simulink model "test_vacc_pkt_10_1"  (Simulink 7.2)
settings: Solver=ode45  StartTime=0.0  StopTime=90000  RelTol=1e-3
libraries: xbsIndex_r4 x802, xps_library x17, casper_library_misc x10, xbsReplacements_r4 x9
(part 1 of 6)
settings Model: Creator=Jason Manley  LastModifiedBy=root
settings OptimizationCC: InitFltsAndDblsToZero=on
settings DebuggingCC: SaveWithParameterizedLinksMsg=none  SignalResolutionControl=TryResolveAllWithWarning  MultiTaskDSMMsg=warning  MultiTaskCondExecSysMsg=none  StrictBusMsg=None
settings RTWCC: IncludeERTFirstTime=on
settings GRTTargetCC: TargetFcnLib=ansi_tfl_tmw.mat

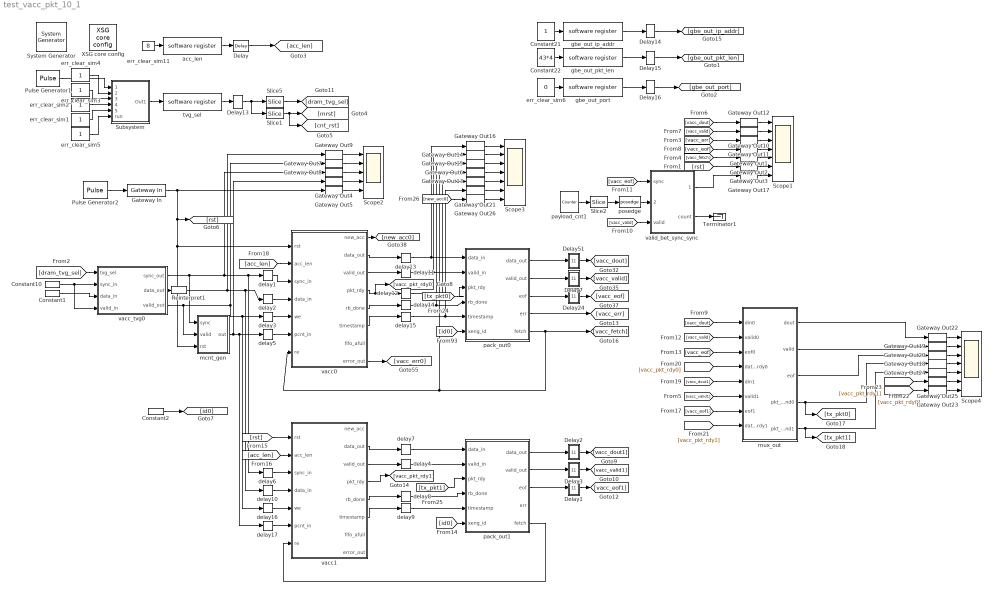
== system test_vacc_pkt_10_1 ==
  " System Generator" : xbsIndex_r4/ System Generator  Tag=genX  SystemSampleTime=-1  xilinxfamily=virtex5  part=xc5vlx110t  speed=-1  package=ff1136  synthesis_tool=XST  clock_wrapper=Clock Enables  directory=./test_vacc_pkt_10_1/sysgen  testbench=off  simulink_period=1  sysclk_period=5  dcm_input_clock_period=100  incr_netlist=off  trim_vbits=Everywhere in SubSystem  dbl_ovrd=According to Block Masks  core_generation=According to Block Masks  run_coregen=off  deprecated_control=off  eval_field=0  block_type=sysgen
      settings: block_version=10.1.3
  Constant1 : xbsIndex_r4/Constant  arith_type=Unsigned  const=0  n_bits=32  bin_pt=0  explicit_period=on  period=1  equ=P=C  opselect=C  inp2=PCIN>>17  opr=+  inp1=P  carry=CIN  dbl_ovrd=off  block_type=constant
  Constant10 : xbsIndex_r4/Constant  arith_type=Boolean  const=0  n_bits=1  bin_pt=0  explicit_period=on  period=1  equ=P=C  opselect=C  inp2=PCIN>>17  opr=+  inp1=P  carry=CIN  dbl_ovrd=off  block_type=constant
  Constant2 : xbsIndex_r4/Constant  arith_type=Unsigned  const=0  n_bits=4  bin_pt=0  explicit_period=on  period=1  equ=P=C  opselect=C  inp2=PCIN>>17  opr=+  inp1=P  carry=CIN  dbl_ovrd=off  block_type=constant
  Constant21 : Constant  OutDataType=sfix(16)  OutScaling=2^0
  Constant22 : Constant  Value=43*4  OutDataType=sfix(16)  OutScaling=2^0
  Delay : xbsIndex_r4/Delay  en=off  latency=1  dbl_ovrd=off  reg_retiming=on  block_type=delay
  Delay1 : Subsystem  AncestorBlock=casper_library/Delays/pipeline  mask(pipeline){latency=2}
      mask help:
      | An explicitly laid-out delay line to avoid mapping to SRL16s
      | for use in pipelining to help achieve timing closure.
      mask init:
      | pipeline_init(gcb, 'latency', latency);
      mask Display:
      | port_label('input', 1, 'd');
      | port_label('output', 1, 'q');
      | disp(['Z^-', num2str(latency)]);
  Delay{13..16} (4 alike) : xbsIndex_r4/Delay  en=off  latency=2  dbl_ovrd=off  reg_retiming=on  block_type=delay
      settings: xl_area=[0, 0, 0, 0, 0, 0, 0]
  Delay2 : Subsystem  AncestorBlock=casper_library/Delays/pipeline  mask(pipeline){latency=2}
      mask help:
      | An explicitly laid-out delay line to avoid mapping to SRL16s
      | for use in pipelining to help achieve timing closure.
      mask init:
      | pipeline_init(gcb, 'latency', latency);
      mask Display:
      | port_label('input', 1, 'd');
      | port_label('output', 1, 'q');
      | disp(['Z^-', num2str(latency)]);
  Delay24 : Subsystem  AncestorBlock=casper_library/Delays/pipeline  mask(pipeline){latency=2}
      mask help:
      | An explicitly laid-out delay line to avoid mapping to SRL16s
      | for use in pipelining to help achieve timing closure.
      mask init:
      | pipeline_init(gcb, 'latency', latency);
      mask Display:
      | port_label('input', 1, 'd');
      | port_label('output', 1, 'q');
      | disp(['Z^-', num2str(latency)]);
  Delay3 : Subsystem  AncestorBlock=casper_library/Delays/pipeline  mask(pipeline){latency=2}
      mask help:
      | An explicitly laid-out delay line to avoid mapping to SRL16s
      | for use in pipelining to help achieve timing closure.
      mask init:
      | pipeline_init(gcb, 'latency', latency);
      mask Display:
      | port_label('input', 1, 'd');
      | port_label('output', 1, 'q');
      | disp(['Z^-', num2str(latency)]);
  Delay51 : Subsystem  AncestorBlock=casper_library/Delays/pipeline  mask(pipeline){latency=2}
      mask help:
      | An explicitly laid-out delay line to avoid mapping to SRL16s
      | for use in pipelining to help achieve timing closure.
      mask init:
      | pipeline_init(gcb, 'latency', latency);
      mask Display:
      | port_label('input', 1, 'd');
      | port_label('output', 1, 'q');
      | disp(['Z^-', num2str(latency)]);
  Delay7 : Subsystem  AncestorBlock=casper_library/Delays/pipeline  mask(pipeline){latency=2}
      mask help:
      | An explicitly laid-out delay line to avoid mapping to SRL16s
      | for use in pipelining to help achieve timing closure.
      mask init:
      | pipeline_init(gcb, 'latency', latency);
      mask Display:
      | port_label('input', 1, 'd');
      | port_label('output', 1, 'q');
      | disp(['Z^-', num2str(latency)]);
  Gateway In : xbsIndex_r4/Gateway In  arith_type=Boolean  n_bits=16  bin_pt=14  quantization="Round  (unbiased: +/- Inf)"  overflow=Saturate  period=1  dbl_ovrd=off  timing_constraint=None  locs_specified=off  LOCs={}  hdl_port=on  block_type=gatewayin
      settings: infoedit="Gateway in block.  Converts inputs of type Simulink integer, double and fixed point to  Xilinx fixed point type.<br><br>Hardware notes:  In hardware these blocks become top level input ports."  block_version=11.4
  Gateway Out{1..26} (26 alike) : xbsIndex_r4/Gateway Out  hdl_port=off  timing_constraint=None  locs_specified=off  LOCs={}  block_type=gatewayout
      settings: infoedit="Gateway out block.  Converts Xilinx fixed point inputs into ouputs of type Simulink integer, double, or fixed point.<P><P>Hardware notes:  In hardware these blocks become top level output ports or are discarded, depending on how they are configured."  xl_area=[0, 0, 0, 0, 0, 0, 0]  block_version=10.1.3
  Pulse Generator1 : DiscretePulseGenerator  Period=4*100*80  PhaseDelay=-4*100*80 + 3
  Pulse Generator2 : DiscretePulseGenerator  Period=8*100*80  PhaseDelay=-2*100*10 + 1
  Reinterpret1 : xbsIndex_r4/Reinterpret  force_arith_type=on  arith_type="Signed  (2's comp)"  force_bin_pt=on  bin_pt=0  block_type=reinterpret
      settings: infoedit="Changes signal type without altering the binary representation.   You can changed the signal between signed and unsigned, and relocate the binary point.<P><P>Hardware notes: In hardware this block costs nothing.<P><P>Example:  Suppose the input is 6 bits wide, signed, with 2 fractional bits, and the output is forced to unsigned with 0 fractional bits.  Then an input of -2.0 (1110.00 in binary 2's complement) becomes an output of 56 (111000 in binary)."  block_version=10.1.3
  Scope1 : Scope  NumInputPorts=7
      settings: YMin=0~0~-1~0~0~0~0  YMax=2.5e+21~1~1~1~1~1~40  SaveName=ScopeData7
  Scope2 : Scope  NumInputPorts=5
      settings: YMin=0~0~0~0~0  YMax=100~1~1~35000~1  SaveName=ScopeData8
  Scope3 : Scope  NumInputPorts=7
      settings: YMin=0~0~0~0~0~0~0  YMax=800~1~1~1~1~17500~1  SaveName=ScopeData10
  Scope4 : Scope  NumInputPorts=7
      settings: YMin=0~0~0~-1~0~-1~0  YMax=1e+19~1~1~1~1~1~1  SaveName=ScopeData11
  Slice1 : xbsIndex_r4/Slice  nbits=1  boolean_output=on  mode=Lower Bit Location + Width  bit1=0  base1=MSB of Input  bit0=31  base0=LSB of Input  dbl_ovrd=off  block_type=slice
      settings: infoedit="Extracts a given range of bits from each input sample and presents it at the output.  The output type is ordinarily unsigned with binary point at zero, but can be Boolean when the slice is one bit wide.<P><P>Hardware notes: In hardware this block costs nothing."  block_version=10.1.3
  Slice2 : xbsIndex_r4/Slice  nbits=1  boolean_output=on  mode=Upper Bit Location + Width  bit1=0  base1=MSB of Input  bit0=1  base0=LSB of Input  dbl_ovrd=off  block_type=slice
      settings: infoedit="Extracts a given range of bits from each input sample and presents it at the output.  The output type is ordinarily unsigned with binary point at zero, but can be Boolean when the slice is one bit wide.<P><P>Hardware notes: In hardware this block costs nothing."  block_version=10.1.3
  Slice5 : xbsIndex_r4/Slice  nbits=6  boolean_output=off  mode=Lower Bit Location + Width  bit1=0  base1=MSB of Input  bit0=9  base0=LSB of Input  dbl_ovrd=off  block_type=slice
      settings: infoedit="Extracts a given range of bits from each input sample and presents it at the output.  The output type is ordinarily unsigned with binary point at zero, but can be Boolean when the slice is one bit wide.<P><P>Hardware notes: In hardware this block costs nothing."  block_version=10.1.3
  Subsystem : Subsystem
  Terminator1 : Terminator
  XSG core config : xps_library/XSG core config  Tag=xps:xsg  SystemSampleTime=-1  hw_sys=iBOB  ibob_linux=off  clk_src=sys_clk  iBOB_clk_src=sys_clk  BEE2_ctrl_clk_src=sys_clk  BEE2_usr_clk_src=sys_clk  ROACH_clk_src=arb_clk  ROACH2_clk_src=adc0_clk  CORR_clk_src=sys_clk  gpio_clk_io_group=iBOB:sma  gpio_clk_bit_index=0  clk_rate=100  sample_period=1  synthesis_tool=XST  mpc_type=powerpc405
  acc_len : xps_library/software register  Tag=xps:sw_reg  SystemSampleTime=-1  io_dir=From Processor  arith_type=Unsigned  bitwidth=32  bin_pt=0  sample_period=1  gw_name=test_vacc_pkt_10_1_acc_len_user_data_out
      link override qdr_vacc_tvg_sel_user_data_out: arith_type=Unsigned  n_bits=32  bin_pt=0  period=1
      link override test_d_v_p_10_1_new_packet_format_acc_len_user_data_out: arith_type=Unsigned  n_bits=32  bin_pt=0  period=1
      link override test_qdr_vacc_acc_len_user_data_out: arith_type=Unsigned  n_bits=32  bin_pt=0  period=1
      link override test_qdr_vacc_tvg_sel_user_data_out: arith_type=Unsigned  n_bits=32  bin_pt=0  period=1
      link override test_vacc_10_1_new_pkt_form_acc_len_user_data_out: arith_type=Unsigned  n_bits=32  bin_pt=0  period=1
      link override test_vacc_pkt_10_1_acc_len_user_data_out: arith_type=Unsigned  n_bits=32  bin_pt=0  period=1
  delay{1..3,5..6,10,16..17} (8 alike) : xbsIndex_r4/Delay  en=off  latency=2  dbl_ovrd=off  reg_retiming=on  block_type=delay
  delay{4,7..9,11..15} (9 alike) : xbsIndex_r4/Delay  en=off  latency=1  dbl_ovrd=off  reg_retiming=on  block_type=delay
  err_clear_sim{1..5} (5 alike) : Constant  OutDataType=sfix(16)  OutScaling=2^0
  err_clear_sim11 : Constant  Value=8  OutDataType=sfix(16)  OutScaling=2^0
  err_clear_sim6 : Constant  Value=0  OutDataType=sfix(16)  OutScaling=2^0
  gbe_out_ip_addr : xps_library/software register  Tag=xps:sw_reg  SystemSampleTime=-1  io_dir=From Processor  arith_type=Unsigned  bitwidth=32  bin_pt=0  sample_period=1  gw_name=test_vacc_pkt_10_1_gbe_out_ip_addr_user_data_out
      link override test_d_v_p_10_1_new_packet_format_gbe_out_ip_addr_user_data_out: arith_type=Unsigned  n_bits=32  bin_pt=0  period=1
      link override test_d_v_p_10_1_new_packet_format_out_ip_addr_user_data_out: arith_type=Unsigned  n_bits=32  bin_pt=0  period=1
      link override test_vacc_10_1_new_pkt_form_gbe_out_ip_addr_user_data_out: arith_type=Unsigned  n_bits=32  bin_pt=0  period=1
      link override test_vacc_pkt_10_1_gbe_out_ip_addr_user_data_out: arith_type=Unsigned  n_bits=32  bin_pt=0  period=1
  gbe_out_pkt_len : xps_library/software register  Tag=xps:sw_reg  SystemSampleTime=-1  io_dir=From Processor  arith_type=Unsigned  bitwidth=32  bin_pt=0  sample_period=1  gw_name=test_vacc_pkt_10_1_gbe_out_pkt_len_user_data_out
      link override test_d_v_p_10_1_new_packet_format_gbe_out_pkt_len_user_data_out: arith_type=Unsigned  n_bits=32  bin_pt=0  period=1
      link override test_d_v_p_10_1_new_packet_format_pkt_len_user_data_out: arith_type=Unsigned  n_bits=32  bin_pt=0  period=1
      link override test_vacc_10_1_new_pkt_form_gbe_out_pkt_len_user_data_out: arith_type=Unsigned  n_bits=32  bin_pt=0  period=1
      link override test_vacc_pkt_10_1_gbe_out_pkt_len_user_data_out: arith_type=Unsigned  n_bits=32  bin_pt=0  period=1
  gbe_out_port : xps_library/software register  Tag=xps:sw_reg  SystemSampleTime=-1  io_dir=From Processor  arith_type=Unsigned  bitwidth=32  bin_pt=0  sample_period=1  gw_name=test_vacc_pkt_10_1_gbe_out_port_user_data_out
      link override test_d_v_p_10_1_new_packet_format_gbe_out_port_user_data_out: arith_type=Unsigned  n_bits=32  bin_pt=0  period=1
      link override test_vacc_10_1_new_pkt_form_gbe_out_port_user_data_out: arith_type=Unsigned  n_bits=32  bin_pt=0  period=1
      link override test_vacc_pkt_10_1_gbe_out_port_user_data_out: arith_type=Unsigned  n_bits=32  bin_pt=0  period=1
  mcnt_gen : Subsystem  mask(sample_and_hold){period=100}
      mask prompts: period "Sample period (clocks)"
      mask help: This block will sample an input signal at a user specified rate and hold the value on the output.
  mux_out : Subsystem  mask{idle_clks=100}
      mask prompts: idle_clks "Rate control. Idle clocks between packets"
      mask init:
      | idle_clks_bits = ceil(log2(idle_clks));
      settings: AttributesFormatString=|
      | Payload Len: 32
      | FIFO latencies: 4.
  pack_out0 : Subsystem  mask(pkt_pack_mask){vector_len=100, heap_len=2000, fifo_latency=2, spead_msw=64, spead_lsw=40, spead_item=6144, pkt_bits=5}
      mask prompts: vector_len "vector length"; heap_len "System heap size"; fifo_latency "Fifo Latency"; spead_msw "SPEAD flavour (MSw)"; spead_lsw "SPEAD flavour (LSw)"; spead_item "SPEAD item number"; pkt_bits "desired payload length (2^?) 64-bit words"
      mask help:
      | This block generates packets from a datastream.
      |
      | Packets are created with a fixed header followed by a user-specified number of 64-bit options.
      |
      | Requires a 64-bit data stream.
      |
      | See the documentation for further details.
      mask init:
      | vector_bits = ceil(log2(vector_len));
      | pkt_len=2^(pkt_bits);
  pack_out1 : Subsystem  mask(pkt_pack_mask){vector_len=100, heap_len=2000, fifo_latency=2, spead_msw=64, spead_lsw=40, spead_item=6144, pkt_bits=5}
      mask prompts: vector_len "vector length"; heap_len "System heap size"; fifo_latency "Fifo Latency"; spead_msw "SPEAD flavour (MSw)"; spead_lsw "SPEAD flavour (LSw)"; spead_item "SPEAD item number"; pkt_bits "desired payload length (2^?) 64-bit words"
      mask help:
      | This block generates packets from a datastream.
      |
      | Packets are created with a fixed header followed by a user-specified number of 64-bit options.
      |
      | Requires a 64-bit data stream.
      |
      | See the documentation for further details.
      mask init:
      | vector_bits = ceil(log2(vector_len));
      | pkt_len=2^(pkt_bits);
  payload_cnt1 : xbsIndex_r4/Counter  cnt_type=Free Running  cnt_to=0  operation=Up  start_count=0  cnt_by_val=1  arith_type=Unsigned  n_bits=12  bin_pt=0  load_pin=off  rst=off  en=off  explicit_period=on  period=1  dbl_ovrd=off  use_behavioral_HDL=off  implementation=Fabric  use_rpm=on  block_type=counter
      settings: xl_area=[0, 0, 0, 0, 0, 0, 0]
  posedge : casper_library_misc/posedge  Tag=Rising Edge Detector  SystemSampleTime=-1
  tvg_sel : xps_library/software register  Tag=xps:sw_reg  SystemSampleTime=-1  io_dir=From Processor  arith_type=Unsigned  bitwidth=32  bin_pt=0  sample_period=1  gw_name=test_vacc_pkt_10_1_tvg_sel_user_data_out
      link override test_d_v_p_10_1_new_packet_format_tvg_sel_user_data_out: arith_type=Unsigned  n_bits=32  bin_pt=0  period=1
      link override test_vacc_10_1_new_pkt_form_tvg_sel_user_data_out: arith_type=Unsigned  n_bits=32  bin_pt=0  period=1
      link override test_vacc_pkt_10_1_tvg_sel_user_data_out: arith_type=Unsigned  n_bits=32  bin_pt=0  period=1
  vacc0 : Subsystem  mask{which_qdr=qdr0, vector_len=100}
      mask prompts: which_qdr "QDR"
      mask help: Hardcoded for X engines with a demux of 8!
      mask init:
      | set_param([gcb, '/qv'], 'which_qdr', which_qdr);
      | fmtstr = sprintf('Vector Length: %d', vector_len);
      | set_param(gcb, 'AttributesFormatString', fmtstr);
      settings: AttributesFormatString=Vector Length: 100
      mask StyleString: popup(qdr0|qdr1),edit
  vacc1 : Subsystem  mask{which_qdr=qdr0, vector_len=100}
      mask prompts: which_qdr "QDR"
      mask help: Hardcoded for X engines with a demux of 8!
      mask init:
      | set_param([gcb, '/qv'], 'which_qdr', which_qdr);
      | fmtstr = sprintf('Vector Length: %d', vector_len);
      | set_param(gcb, 'AttributesFormatString', fmtstr);
      settings: AttributesFormatString=Vector Length: 100
      mask StyleString: popup(qdr0|qdr1),edit
  vacc_tvg0 : Subsystem  AncestorBlock=casper_library/Accumulators/vacc_tvg  mask{len=100}
      mask prompts: len "Number of Vectors"
      mask init:
      | fmtstr = sprintf('Vector Length: %d', len);
      | set_param(gcb, 'AttributesFormatString', fmtstr);
      settings: AttributesFormatString=Vector Length: 100
  valid_bet_sync_sync : Subsystem
  wires:
  tvg_sel/1 -> Delay13/1
  Slice5/1 -> [dram_tvg_sel]
  err_clear_sim1/1 -> Subsystem/5(data_sel)
  err_clear_sim2/1 -> Subsystem/4(valid_sel)
  err_clear_sim3/1 -> Subsystem/3(inj_vector)
  err_clear_sim4/1 -> Subsystem/2(inj_counter)
  Subsystem/1(Out1) -> tvg_sel/1
  Pulse Generator1/1 -> Subsystem/1(new_acc)
  err_clear_sim5/1 -> Subsystem/6(run)
  Constant22/1 -> gbe_out_pkt_len/1
  Constant21/1 -> gbe_out_ip_addr/1
  gbe_out_ip_addr/1 -> Delay14/1
  gbe_out_pkt_len/1 -> Delay15/1
  Slice1/1 -> [mrst], [cnt_rst]
  acc_len/1 -> Delay/1
  err_clear_sim11/1 -> acc_len/1
  err_clear_sim6/1 -> gbe_out_port/1
  gbe_out_port/1 -> Delay16/1
  Delay13/1 -> Slice5/1, Slice1/1
  Delay14/1 -> [gbe_out_ip_addr]
  Delay15/1 -> [gbe_out_pkt_len]
  Delay16/1 -> [gbe_out_port]
  pack_out0/3(eof) -> Delay24/1(d)
  pack_out0/1(data_out) -> Delay51/1(d)
  pack_out0/2(valid_out) -> Delay7/1(d)
  Gateway In/1 -> Gateway Out5/1, mcnt_gen/3(rst), vacc0/1(rst), [rst]
  Delay51/1(q) -> [vacc_dout]
  Delay7/1(q) -> [vacc_valid]
  Delay24/1(q) -> [vacc_eof]
  vacc_tvg0/1(sync_out) -> Gateway Out8/1, delay1/1, delay6/1, mcnt_gen/1(sync)
  vacc_tvg0/2(data_out) -> Reinterpret1/1
  vacc_tvg0/3(valid_out) -> Gateway Out7/1, delay3/1, delay16/1, mcnt_gen/2(valid)
  Reinterpret1/1 -> Gateway Out9/1, delay2/1, delay10/1
  Delay/1 -> [acc_len]
  [dram_tvg_sel] -> vacc_tvg0/1(tvg_sel)
  Constant10/1 -> vacc_tvg0/2(sync_in), vacc_tvg0/4(valid_in)
  Constant1/1 -> vacc_tvg0/3(data_in)
  Gateway Out5/1 -> Scope2/5
  Gateway Out4/1 -> Scope2/4
  Gateway Out9/1 -> Scope2/1
  Gateway Out7/1 -> Scope2/2
  Gateway Out8/1 -> Scope2/3
  Gateway Out3/1 -> Scope1/6
  Gateway Out2/1 -> Scope1/5
  Gateway Out1/1 -> Scope1/4
  Gateway Out12/1 -> Scope1/1
  Gateway Out10/1 -> Scope1/2
  Gateway Out11/1 -> Scope1/3
  [vacc_dout] -> Gateway Out12/1
  [vacc_valid] -> Gateway Out10/1
  [vacc_eof] -> Gateway Out1/1
  Gateway Out13/1 -> Scope3/5
  Gateway Out6/1 -> Scope3/4
  Gateway Out16/1 -> Scope3/1
  Gateway Out14/1 -> Scope3/2
  Gateway Out15/1 -> Scope3/3
  valid_bet_sync_sync/2(count) -> Terminator1/1
  [vacc_valid] -> valid_bet_sync_sync/3(valid)
  [vacc_eof] -> valid_bet_sync_sync/1(sync)
  payload_cnt1/1 -> Slice2/1
  Slice2/1 -> posedge/1
  Gateway Out17/1 -> Scope1/7
  posedge/1 -> valid_bet_sync_sync/2(rst_max)
  valid_bet_sync_sync/1(max_count) -> Gateway Out17/1
  mcnt_gen/1(out) -> Gateway Out4/1, delay5/1, delay17/1
  Pulse Generator2/1 -> Gateway In/1
  Gateway Out21/1 -> Scope3/6
  vacc0/1(new_acc) -> [new_acc0]
  vacc0/6(timestamp) -> delay15/1
  vacc0/8(error_out) -> [vacc_err0]
  vacc0/2(data_out) -> delay13/1
  vacc0/3(valid_out) -> delay11/1
  vacc0/5(rb_done) -> delay14/1
  vacc0/4(pkt_rdy) -> [vacc_pkt_rdy0], delay12/1
  [id0] -> pack_out0/6(xeng_id)
  pack_out0/5(fetch) -> vacc0/7(re), Gateway Out6/1, [vacc_fetch]
  delay13/1 -> Gateway Out16/1, pack_out0/1(data_in)
  delay11/1 -> Gateway Out14/1, pack_out0/2(valid_in)
  delay12/1 -> Gateway Out13/1
  delay14/1 -> Gateway Out15/1, pack_out0/4(rb_done)
  delay15/1 -> Gateway Out21/1, pack_out0/5(timestamp)
  delay5/1 -> vacc0/6(pcnt_in)
  [acc_len] -> vacc0/2(acc_len)
  delay1/1 -> vacc0/3(sync_in)
  delay2/1 -> vacc0/4(data_in)
  delay3/1 -> vacc0/5(we)
  [rst] -> Gateway Out3/1
  Constant2/1 -> [id0]
  pack_out1/3(eof) -> Delay1/1(d)
  pack_out1/1(data_out) -> Delay2/1(d)
  pack_out1/2(valid_out) -> Delay3/1(d)
  Delay2/1(q) -> [vacc_dout1]
  Delay3/1(q) -> [vacc_valid1]
  Delay1/1(q) -> [vacc_eof1]
  vacc1/6(timestamp) -> delay9/1
  vacc1/2(data_out) -> delay7/1
  vacc1/3(valid_out) -> delay4/1
  vacc1/5(rb_done) -> delay8/1
  vacc1/4(pkt_rdy) -> [vacc_pkt_rdy1]
  [id0] -> pack_out1/6(xeng_id)
  pack_out1/5(fetch) -> vacc1/7(re)
  delay7/1 -> pack_out1/1(data_in)
  delay4/1 -> pack_out1/2(valid_in)
  delay8/1 -> pack_out1/4(rb_done)
  delay9/1 -> pack_out1/5(timestamp)
  [rst] -> vacc1/1(rst)
  [acc_len] -> vacc1/2(acc_len)
  pack_out0/4(err) -> [vacc_err]
  [vacc_fetch] -> Gateway Out2/1
  [vacc_err] -> Gateway Out11/1
  [vacc_dout] -> mux_out/1(din0)
  [vacc_valid] -> mux_out/2(valid0)
  [vacc_eof] -> mux_out/3(eof0)
  [vacc_pkt_rdy0] -> mux_out/4(data_rdy0)
  [vacc_dout1] -> mux_out/5(din1)
  [vacc_valid1] -> mux_out/6(valid1)
  [vacc_eof1] -> mux_out/7(eof1)
  [vacc_pkt_rdy1] -> mux_out/8(data_rdy1)
  Gateway Out25/1 -> Scope4/6
  Gateway Out24/1 -> Scope4/5
  Gateway Out18/1 -> Scope4/4
  Gateway Out22/1 -> Scope4/1
  Gateway Out19/1 -> Scope4/2
  Gateway Out20/1 -> Scope4/3
  mux_out/1(dout) -> Gateway Out22/1
  mux_out/2(valid) -> Gateway Out19/1
  Gateway Out23/1 -> Scope4/7
  mux_out/3(eof) -> Gateway Out20/1
  mux_out/4(pkt_send0) -> Gateway Out18/1, [tx_pkt0]
  mux_out/5(pkt_send1) -> Gateway Out24/1, [tx_pkt1]
  [vacc_pkt_rdy0] -> Gateway Out25/1
  [vacc_pkt_rdy1] -> Gateway Out23/1
  [tx_pkt0] -> pack_out0/3(pkt_rdy)
  [tx_pkt1] -> pack_out1/3(pkt_rdy)
  delay6/1 -> vacc1/3(sync_in)
  delay10/1 -> vacc1/4(data_in)
  delay16/1 -> vacc1/5(we)
  delay17/1 -> vacc1/6(pcnt_in)
  Gateway Out26/1 -> Scope3/7
  [new_acc0] -> Gateway Out26/1

== system test_vacc_pkt_10_1/Delay1 ==
  d : Inport
  Register0 : xbsIndex_r4/Register  init=0  rst=off  en=off  dbl_ovrd=off  block_type=register
  Register1 : xbsIndex_r4/Register  init=0  rst=off  en=off  dbl_ovrd=off  block_type=register
  q : Outport
  wires:
  Register0/1 -> Register1/1
  d/1 -> Register0/1
  Register1/1 -> q/1

== system test_vacc_pkt_10_1/Delay2 ==
  d : Inport
  Register0 : xbsIndex_r4/Register  init=0  rst=off  en=off  dbl_ovrd=off  block_type=register
  Register1 : xbsIndex_r4/Register  init=0  rst=off  en=off  dbl_ovrd=off  block_type=register
  q : Outport
  wires:
  Register0/1 -> Register1/1
  d/1 -> Register0/1
  Register1/1 -> q/1

== system test_vacc_pkt_10_1/Delay24 ==
  d : Inport
  Register0 : xbsIndex_r4/Register  init=0  rst=off  en=off  dbl_ovrd=off  block_type=register
  Register1 : xbsIndex_r4/Register  init=0  rst=off  en=off  dbl_ovrd=off  block_type=register
  q : Outport
  wires:
  Register0/1 -> Register1/1
  d/1 -> Register0/1
  Register1/1 -> q/1

== system test_vacc_pkt_10_1/Delay3 ==
  d : Inport
  Register0 : xbsIndex_r4/Register  init=0  rst=off  en=off  dbl_ovrd=off  block_type=register
  Register1 : xbsIndex_r4/Register  init=0  rst=off  en=off  dbl_ovrd=off  block_type=register
  q : Outport
  wires:
  Register0/1 -> Register1/1
  d/1 -> Register0/1
  Register1/1 -> q/1

== system test_vacc_pkt_10_1/Delay51 ==
  d : Inport
  Register0 : xbsIndex_r4/Register  init=0  rst=off  en=off  dbl_ovrd=off  block_type=register
  Register1 : xbsIndex_r4/Register  init=0  rst=off  en=off  dbl_ovrd=off  block_type=register
  q : Outport
  wires:
  Register0/1 -> Register1/1
  d/1 -> Register0/1
  Register1/1 -> q/1

== system test_vacc_pkt_10_1/Delay7 ==
  d : Inport
  Register0 : xbsIndex_r4/Register  init=0  rst=off  en=off  dbl_ovrd=off  block_type=register
  Register1 : xbsIndex_r4/Register  init=0  rst=off  en=off  dbl_ovrd=off  block_type=register
  q : Outport
  wires:
  Register0/1 -> Register1/1
  d/1 -> Register0/1
  Register1/1 -> q/1

== system test_vacc_pkt_10_1/Subsystem ==
  new_acc : Inport  OutDataType=sfix(16)  OutScaling=2^0
  inj_counter : Inport  Port=2  OutDataType=sfix(16)  OutScaling=2^0
  inj_vector : Inport  Port=3  OutDataType=sfix(16)  OutScaling=2^0
  valid_sel : Inport  Port=4  OutDataType=sfix(16)  OutScaling=2^0
  data_sel : Inport  Port=5  OutDataType=sfix(16)  OutScaling=2^0
  run : Inport  Port=6  OutDataType=sfix(16)  OutScaling=2^0
  Sum : Sum  Inputs=|++++++  OutDataType=sfix(16)  OutScaling=2^0
  data_sel1 : Subsystem  mask{bit_pos=10}
      mask prompts: bit_pos "bit position"
  inj_counter1 : Subsystem  mask{bit_pos=13}
      mask prompts: bit_pos "bit position"
  inj_vector1 : Subsystem  mask{bit_pos=12}
      mask prompts: bit_pos "bit position"
  new_acc2 : Subsystem  mask{bit_pos=14}
      mask prompts: bit_pos "bit position"
  run1 : Subsystem  mask{bit_pos=9}
      mask prompts: bit_pos "bit position"
  valid_sel1 : Subsystem  mask{bit_pos=11}
      mask prompts: bit_pos "bit position"
  Out1 : Outport  OutDataType=sfix(16)  OutScaling=2^0
  wires:
  new_acc2/1(Out1) -> Sum/1
  inj_counter1/1(Out1) -> Sum/2
  inj_vector1/1(Out1) -> Sum/3
  valid_sel1/1(Out1) -> Sum/4
  data_sel1/1(Out1) -> Sum/5
  run1/1(Out1) -> Sum/6
  new_acc/1 -> new_acc2/1(In1)
  inj_counter/1 -> inj_counter1/1(In1)
  inj_vector/1 -> inj_vector1/1(In1)
  valid_sel/1 -> valid_sel1/1(In1)
  Sum/1 -> Out1/1
  data_sel/1 -> data_sel1/1(In1)
  run/1 -> run1/1(In1)

== system test_vacc_pkt_10_1/mcnt_gen ==
  sync : Inport
  valid : Inport  Port=2
  rst : Inport  Port=3
  Constant3 : xbsIndex_r4/Constant  arith_type=Unsigned  const=period-1  n_bits=ceil(log2(period))  bin_pt=0  explicit_period=on  period=1  equ=P=C  opselect=C  inp2=PCIN>>17  opr=+  inp1=P  carry=CIN  dbl_ovrd=off  block_type=constant
  Counter : xbsIndex_r4/Counter  cnt_type=Free Running  cnt_to=1  operation=Up  start_count=0  cnt_by_val=1  arith_type=Unsigned  n_bits=40  bin_pt=0  load_pin=off  rst=on  en=on  explicit_period=on  period=1  dbl_ovrd=off  use_behavioral_HDL=off  implementation=Fabric  use_rpm=on  block_type=counter
      settings: xl_area=[0, 0, 0, 0, 0, 0, 0]
  Counter4 : xbsIndex_r4/Counter  cnt_type=Free Running  cnt_to=Inf  operation=Up  start_count=0  cnt_by_val=1  arith_type=Unsigned  n_bits=ceil(log2(period))  bin_pt=0  load_pin=off  rst=on  en=on  explicit_period=on  period=1  dbl_ovrd=off  use_behavioral_HDL=off  implementation=Fabric  use_rpm=on  block_type=counter
      settings: xl_area=[0, 0, 0, 0, 0, 0, 0]
  Logical : xbsIndex_r4/Logical  logical_function=OR  inputs=2  en=off  latency=0  precision=Full  arith_type=Unsigned  n_bits=16  bin_pt=0  align_bp=on  dbl_ovrd=off  block_type=logical
  Relational : xbsIndex_r4/Relational  mode=a>=b  en=off  latency=0  dbl_ovrd=off  block_type=relational
      settings: xl_area=[0, 0, 0, 0, 0, 0, 0]  block_version=10.1.3
  mcnt_reg1 : xbsIndex_r4/Register  init=0  rst=on  en=on  dbl_ovrd=off  block_type=register
  out : Outport
  wires:
  valid/1 -> Counter4/2, Counter/2
  Relational/1 -> Logical/1
  Constant3/1 -> Relational/2
  Counter4/1 -> Relational/1
  Logical/1 -> Counter4/1
  sync/1 -> Logical/2, mcnt_reg1/2
  Counter/1 -> out/1
  rst/1 -> mcnt_reg1/1, mcnt_reg1/3
  mcnt_reg1/1 -> Counter/1

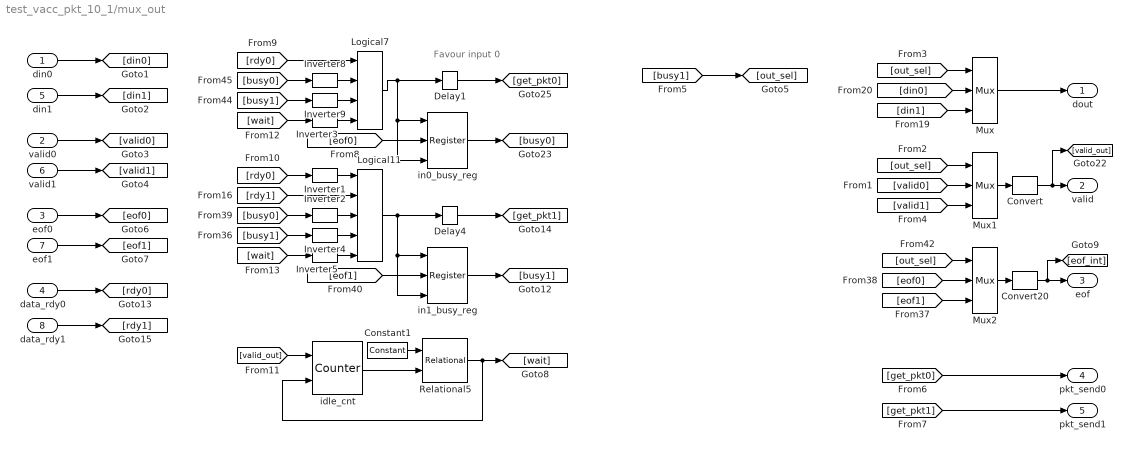
== system test_vacc_pkt_10_1/mux_out ==
  note: Favour input 0
  din0 : Inport  OutDataType=sfix(16)  OutScaling=2^0
  valid0 : Inport  Port=2  OutDataType=sfix(16)  OutScaling=2^0
  eof0 : Inport  Port=3  OutDataType=sfix(16)  OutScaling=2^0
  data_rdy0 : Inport  Port=4  OutDataType=sfix(16)  OutScaling=2^0
  din1 : Inport  Port=5  OutDataType=sfix(16)  OutScaling=2^0
  valid1 : Inport  Port=6  OutDataType=sfix(16)  OutScaling=2^0
  eof1 : Inport  Port=7  OutDataType=sfix(16)  OutScaling=2^0
  data_rdy1 : Inport  Port=8  OutDataType=sfix(16)  OutScaling=2^0
  Constant1 : xbsIndex_r4/Constant  arith_type=Unsigned  const=idle_clks  n_bits=idle_clks_bits+1  bin_pt=0  explicit_period=on  period=1  equ=P=C  opselect=C  inp2=PCIN>>17  opr=+  inp1=P  carry=CIN  dbl_ovrd=off  block_type=constant
  Convert : xbsIndex_r4/Convert  arith_type=Boolean  n_bits=8  bin_pt=6  quantization=Truncate  overflow=Wrap  latency=0  dbl_ovrd=off  pipeline=off  block_type=convert
      settings: xl_area=[0, 0, 0, 0, 0, 0, 0]  block_version=10.1.3
  Convert20 : xbsIndex_r4/Convert  arith_type=Boolean  n_bits=8  bin_pt=6  quantization=Truncate  overflow=Wrap  latency=0  dbl_ovrd=off  pipeline=off  block_type=convert
      settings: xl_area=[0, 0, 0, 0, 0, 0, 0]  block_version=10.1.3
  Delay1 : xbsIndex_r4/Delay  en=off  latency=1  dbl_ovrd=off  reg_retiming=on  block_type=delay
      settings: xl_area=[0, 0, 0, 0, 0, 0, 0]
  Delay4 : xbsIndex_r4/Delay  en=off  latency=1  dbl_ovrd=off  reg_retiming=on  block_type=delay
      settings: xl_area=[0, 0, 0, 0, 0, 0, 0]
  Inverter{1..5,8..9} (7 alike) : xbsIndex_r4/Inverter  en=off  latency=0  dbl_ovrd=off  block_type=inv
      settings: xl_area=[0, 0, 0, 0, 0, 0, 0]
  Logical11 : xbsIndex_r4/Logical  logical_function=AND  inputs=5  en=off  latency=0  precision=Full  arith_type=Unsigned  n_bits=8  bin_pt=2  align_bp=on  dbl_ovrd=off  block_type=logical
      settings: xl_area=[0, 0, 0, 0, 0, 0, 0]
  Logical7 : xbsIndex_r4/Logical  logical_function=AND  inputs=4  en=off  latency=0  precision=Full  arith_type=Unsigned  n_bits=8  bin_pt=2  align_bp=on  dbl_ovrd=off  block_type=logical
      settings: xl_area=[0, 0, 0, 0, 0, 0, 0]
  Mux : xbsIndex_r4/Mux  inputs=2  en=off  latency=0  precision=Full  arith_type="Signed  (2's comp)"  n_bits=8  bin_pt=2  quantization=Truncate  overflow=Wrap  dbl_ovrd=off  block_type=mux
      settings: xl_area=[0, 0, 0, 0, 0, 0, 0]
  Mux1 : xbsIndex_r4/Mux  inputs=2  en=off  latency=0  precision=Full  arith_type="Signed  (2's comp)"  n_bits=8  bin_pt=2  quantization=Truncate  overflow=Wrap  dbl_ovrd=off  block_type=mux
      settings: xl_area=[0, 0, 0, 0, 0, 0, 0]
  Mux2 : xbsIndex_r4/Mux  inputs=2  en=off  latency=0  precision=Full  arith_type="Signed  (2's comp)"  n_bits=8  bin_pt=2  quantization=Truncate  overflow=Wrap  dbl_ovrd=off  block_type=mux
      settings: xl_area=[0, 0, 0, 0, 0, 0, 0]
  Relational5 : xbsIndex_r4/Relational  mode=a>=b  en=off  latency=1  dbl_ovrd=off  block_type=relational
      settings: xl_area=[0, 0, 0, 0, 0, 0, 0]  block_version=10.1.3
  idle_cnt : xbsIndex_r4/Counter  cnt_type=Free Running  cnt_to=Inf  operation=Up  start_count=0  cnt_by_val=1  arith_type=Unsigned  n_bits=idle_clks_bits+1  bin_pt=0  load_pin=off  rst=on  en=on  explicit_period=on  period=1  dbl_ovrd=off  use_behavioral_HDL=off  implementation=Fabric  use_rpm=on  block_type=counter
      settings: xl_area=[0, 0, 0, 0, 0, 0, 0]
  in0_busy_reg : xbsIndex_r4/Register  init=0  rst=on  en=on  dbl_ovrd=off  block_type=register
      settings: xl_area=[0, 0, 0, 0, 0, 0, 0]
  in1_busy_reg : xbsIndex_r4/Register  init=0  rst=on  en=on  dbl_ovrd=off  block_type=register
      settings: xl_area=[0, 0, 0, 0, 0, 0, 0]
  dout : Outport  OutDataType=sfix(16)  OutScaling=2^0
  valid : Outport  Port=2  OutDataType=sfix(16)  OutScaling=2^0
  eof : Outport  Port=3  OutDataType=sfix(16)  OutScaling=2^0
  pkt_send0 : Outport  Port=4  OutDataType=sfix(16)  OutScaling=2^0
  pkt_send1 : Outport  Port=5  OutDataType=sfix(16)  OutScaling=2^0
  wires:
  Mux/1 -> dout/1
  Mux1/1 -> Convert/1
  Mux2/1 -> Convert20/1
  Convert/1 -> valid/1, [valid_out]
  [out_sel] -> Mux/1
  [out_sel] -> Mux2/1
  [out_sel] -> Mux1/1
  Convert20/1 -> [eof_int], eof/1
  [din0] -> Mux/2
  [din1] -> Mux/3
  [eof0] -> Mux2/2
  [eof1] -> Mux2/3
  din0/1 -> [din0]
  din1/1 -> [din1]
  valid0/1 -> [valid0]
  valid1/1 -> [valid1]
  eof0/1 -> [eof0]
  eof1/1 -> [eof1]
  data_rdy0/1 -> [rdy0]
  data_rdy1/1 -> [rdy1]
  [valid0] -> Mux1/2
  [valid1] -> Mux1/3
  [eof0] -> in0_busy_reg/2
  Logical7/1 -> in0_busy_reg/1, in0_busy_reg/3, Delay1/1
  [rdy0] -> Logical7/1
  Inverter8/1 -> Logical7/2
  [busy0] -> Inverter8/1
  [busy1] -> Inverter9/1
  Inverter9/1 -> Logical7/3
  [eof1] -> in1_busy_reg/2
  Logical11/1 -> in1_busy_reg/3, in1_busy_reg/1, Delay4/1
  [rdy1] -> Logical11/2
  in1_busy_reg/1 -> [busy1]
  Inverter2/1 -> Logical11/3
  [busy0] -> Inverter2/1
  [busy1] -> Inverter4/1
  Inverter4/1 -> Logical11/4
  [get_pkt0] -> pkt_send0/1
  [get_pkt1] -> pkt_send1/1
  [busy1] -> [out_sel]
  in0_busy_reg/1 -> [busy0]
  Inverter1/1 -> Logical11/1
  [rdy0] -> Inverter1/1
  [valid_out] -> idle_cnt/1
  idle_cnt/1 -> Relational5/2
  Constant1/1 -> Relational5/1
  Relational5/1 -> idle_cnt/2, [wait]
  Inverter3/1 -> Logical7/4
  [wait] -> Inverter3/1
  Inverter5/1 -> Logical11/5
  [wait] -> Inverter5/1
  Delay4/1 -> [get_pkt1]
  Delay1/1 -> [get_pkt0]
